simulink model "Freq_Estimation_IeI"  (R2021a)
settings: Solver=VariableStepAuto  StartTime=0.0  StopTime=10000  RelTol=1e-3
settings Model: Creator=valerio  LastModifiedBy=simon

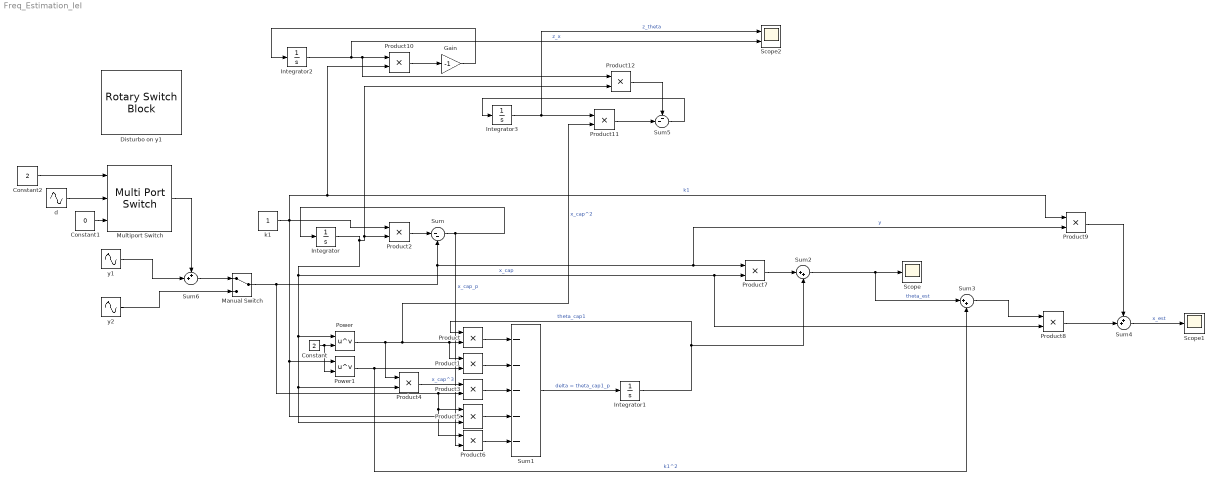
== system Freq_Estimation_IeI ==
  Constant : Constant  Value=2
  Constant1 : Constant  Value=0
  Constant2 : Constant  Value=2
  Disturbo on y1 : RotarySwitchBlock  LabelPosition=Hide
      settings: Values={{'Off', 'On'}, [2 1]}
  Gain : Gain  Gain=-1
  Integrator : Integrator
  Integrator1 : Integrator
  Integrator2 : Integrator  InitialCondition=1
  Integrator3 : Integrator  InitialCondition=1
  Manual Switch : ManualSwitch
  Multiport Switch : MultiPortSwitch  Inputs=2
  Power : Math  Operator=pow  SaturateOnIntegerOverflow=on
  Power1 : Math  Operator=pow  SaturateOnIntegerOverflow=on
  Product{,1..4,6..12} (12 alike) : Product
  Product5 : Product  Inputs=3
  Scope : Scope
  Scope1 : Scope
  Scope2 : Scope  NumInputPorts=2
  Sum : Sum  Inputs=|--
  Sum1 : Sum  Inputs=-----
  Sum2 : Sum  Inputs=|++
  Sum3 : Sum  Inputs=|++
  Sum4 : Sum  Inputs=++|
  Sum5 : Sum  Inputs=--|
  Sum6 : Sum  Inputs=++|
  d : Sin  Amplitude=0.001  Frequency=50  SampleTime=0
  k1 : Constant
  y1 : Sin  Frequency=100  SampleTime=0
  y2 : Sin  SampleTime=0
  wires:
  y2/1 -> Manual Switch/2
  Integrator/1 -> Product12/2, Product2/2, Product8/2, Product7/2, Product5/3, Product4/2, Power/1  "x_cap"
  Manual Switch/1 -> Product6/1, Product5/1, Product3/2, Sum/2, Product9/2, Product7/1  "y"
  Sum/1 -> Product6/2, Integrator/1  "x_cap_p"
  Sum1/1 -> Integrator1/1  "delta = theta_cap1_p"
  Integrator1/1 -> Sum2/2, Product/1  "theta_cap1"
  Power/1 -> Product4/1, Product11/2, Product1/1, Product/2  "x_cap^2"
  Constant/1 -> Power1/2, Power/2
  Product/1 -> Sum1/1
  Product2/1 -> Sum/1
  k1/1 -> Product5/2, Power1/1, Product9/1, Product10/2, Product2/1  "k1"
  Power1/1 -> Sum3/2, Product1/2  "k1^2"
  Product1/1 -> Sum1/2
  Product3/1 -> Sum1/3
  Product4/1 -> Product3/1  "x_cap^3"
  Product5/1 -> Sum1/4
  Product7/1 -> Sum2/1
  Sum2/1 -> Sum3/1, Scope/1  "theta_est"
  Sum3/1 -> Product8/1
  Product8/1 -> Sum4/2
  Product9/1 -> Sum4/1
  Sum4/1 -> Scope1/1  "x_est"
  Product6/1 -> Sum1/5
  Integrator2/1 -> Scope2/2, Product12/1, Product10/1  "z_x"
  Product10/1 -> Gain/1
  Gain/1 -> Integrator2/1
  Product11/1 -> Sum5/2
  Integrator3/1 -> Scope2/1, Product11/1  "z_theta"
  Product12/1 -> Sum5/1
  Sum5/1 -> Integrator3/1
  Sum6/1 -> Manual Switch/1
  y1/1 -> Sum6/2
  d/1 -> Multiport Switch/2
  Constant1/1 -> Multiport Switch/3
  Constant2/1 -> Multiport Switch/1
  Multiport Switch/1 -> Sum6/1
